simulink model "p2_e_sim"  (R2019a)
settings: Solver=VariableStepAuto  StartTime=0.0  StopTime=200  RelTol=1e-3
values from neighbouring files (symbols this model uses):
  A = [-0.322 0.052 0.028 -1.12   0.002 ... (first row only)    [p1.m]    (also in p2_e.m)
  B = [ 0; 0; 0; 0; 7.5]    [p2_e.m]
  C = [ 1 0 0 0 0 ... (first row only)    [p2_e.m]
  D = [ 0; 0; 0; 0]    [p2_e.m]
  k_dphi = k_d_phi    [p2_d.m]    (also in p2_e.m)
  k_ix = k_i_chi    [p2_d.m]    (also in p2_e.m)
  k_pphi = k_p_phi    [p2_d.m]    (also in p2_e.m)
  k_px = k_p_chi    [p2_d.m]    (also in p2_e.m)
undefined symbols (not defined in the file or in its folder): sigbuilder_block
libraries: simulink_extras x4
settings Model: Creator=lenovo  LastModifiedBy=zhy

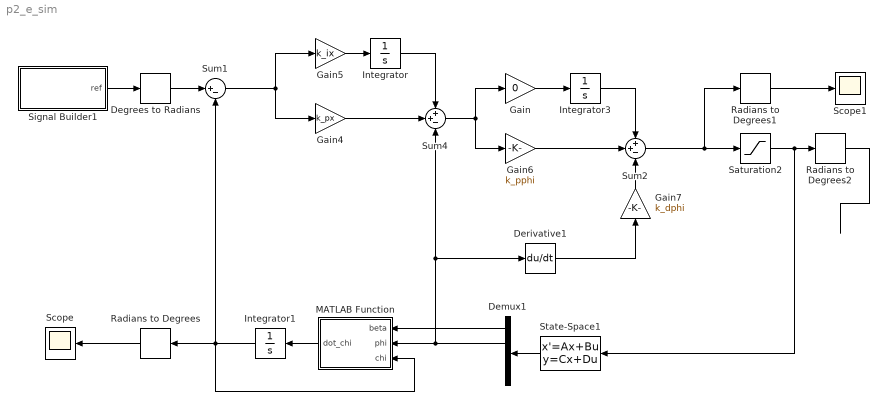
== system p2_e_sim ==
  Degrees to Radians : simulink_extras/Transformations/Degrees to Radians
  Demux1 : Demux
  Derivative1 : Derivative
  Gain : Gain  Gain=0
  Gain4 : Gain  Gain=k_px
  Gain5 : Gain  Gain=k_ix
  Gain6 : Gain  Gain=k_pphi
  Gain7 : Gain  Gain=k_dphi
  Integrator : Integrator
  Integrator1 : Integrator
  Integrator3 : Integrator
  MATLAB Function : MATLAB Function  TreatAsAtomicUnit=on
  Radians to Degrees : simulink_extras/Transformations/Radians to Degrees
  Radians to Degrees1 : simulink_extras/Transformations/Radians to Degrees
  Radians to Degrees2 : simulink_extras/Transformations/Radians to Degrees
  Saturation2 : Saturate  UpperLimit=30*deg2rad  LowerLimit=-30*deg2rad
  Scope : Scope
  Scope1 : Scope
  Signal Builder1 : Subsystem  Tag=STV Subsys  LoadFcn=sigbuilder_block('load');  StartFcn=sigbuilder_block('start');  StopFcn=sigbuilder_block('stop');  ClipboardFcn=sigbuilder_block('clipboard');  mask(Sigbuilder block){tuvar=[0:10]}
      mask help: Simulink:masks:SigbuilderBlock_MD
      mask init:
      | if ~strcmp(get_param(bdroot(gcbh),'SimulationStatus'),'stopped') tuvar = sigbuilder_block('maskInit'); end
      settings: CopyFcn=sigbuilder_block('copy');  DeleteFcn=sigbuilder_block('delete');  ModelCloseFcn=sigbuilder_block('modelClose');  PreSaveFcn=sigbuilder_block('preSave');  PauseFcn=sigbuilder_block('pause');  ContinueFcn=sigbuilder_block('continue');  NameChangeFcn=sigbuilder_block('namechange');  OpenFcn=sigbuilder_block('open',[411 163.2 550.8 400.2 ]);  CloseFcn=sigbuilder_block('close');
      mask Display: plot(0, 0, 100, 100,[2, 2, 32, 32, 2], [68, 8, 8, 68, 68],[32, 2], [38, 38], [32, 19, 2],[53, 60, 44], [32, 17, 17, 2],[16, 16, 31, 31]);txt = getActiveGroup(gcbh);text(2, 100, txt,'verticalAlignment', 'top');
  State-Space1 : StateSpace  A=A  B=B  C=C  D=D  InitialCondition=0
  Sum1 : Sum  Inputs=|+-
  Sum2 : Sum  Inputs=++-
  Sum4 : Sum  Inputs=++-
  wires:
  Saturation2/1 -> Radians to Degrees2/1, State-Space1/1
  State-Space1/1 -> Demux1/1
  MATLAB Function/1(dot_chi) -> Integrator1/1
  Integrator1/1 -> Radians to Degrees/1, MATLAB Function/3(chi), Sum1/2
  Gain6/1 -> Sum2/2
  Gain5/1 -> Integrator/1
  Gain/1 -> Integrator3/1
  Sum4/1 -> Gain6/1, Gain/1
  Sum1/1 -> Gain4/1, Gain5/1
  Gain7/1 -> Sum2/3
  Gain4/1 -> Sum4/2
  Integrator3/1 -> Sum2/1
  Demux1/2 -> MATLAB Function/2(phi), Sum4/3, Derivative1/1
  Derivative1/1 -> Gain7/1
  Demux1/1 -> MATLAB Function/1(beta)
  Signal Builder1/1(ref) -> Degrees to Radians/1
  Degrees to Radians/1 -> Sum1/1
  Radians to Degrees/1 -> Scope/1
  Sum2/1 -> Radians to Degrees1/1, Saturation2/1
  Radians to Degrees1/1 -> Scope1/1
  Integrator/1 -> Sum4/1
  Radians to Degrees2/1 -> ?

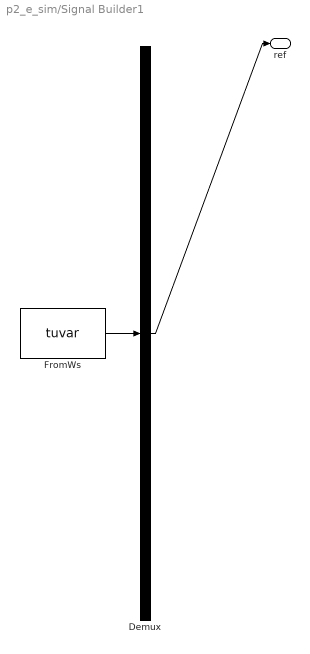
== system p2_e_sim/Signal Builder1 ==
  Demux : Demux  Tag=STV Demux  Outputs=1
  FromWs : FromWorkspace  Tag=STV FromWs  VariableName=tuvar  SampleTime=0
      SigBuilderData=|
      | common.afterFinalStr = 'Extrapolate'
      | common.sampleTime = 0
      | dataSet.timeRange = [0 200]
      | dataSet.name = 'Group 1'
      | sbobj.Groups.Name = 'Group 1'
      | sbobj.Groups.Signals.Name = 'ref'
      | sbobj.Groups.Signals.XData = [0 25 25 75 75 125 125 200]
      | sbobj.Groups.Signals.YData = [0 0 5 5 10 10 15 15]
      | sbobj.Groups.TimeRange = [0 200]
  ref : Outport  Tag=STV Outport
  wires:
  FromWs/1 -> Demux/1
  Demux/1 -> ref/1

== matlab function p2_e_sim/MATLAB Function ==
  data: beta input; phi input; dot_chi output; chi input
function dot_chi = fcn(beta,phi,chi)
psi = chi-beta;
g = 9.81;
V_a = 580/3.6;
V_g = V_a;
d = 1.5*pi/180; %bias
dot_chi = g/V_g*tan(phi+d)*cos(chi-psi);
